simulink model "Dfig2014a"  (R2016a)
settings: Solver=ode45  StartTime=0.0  StopTime=1  RelTol=1e-3
values from neighbouring files (symbols this model uses):
  beta = beta (k)    [Parameter_2M_DFIG.m]    (also in Parameter_2M_DFIG_GSC.m)
  Cbus = 80e-3    (= 0.08)    [Parameter_2M_DFIG.m]    (also in Parameter_2M_DFIG_GSC.m; ini2.m; init.m)
  Cbus_bess = 15e-3    (= 0.015)    [Parameter_2M_DFIG.m]    (also in Parameter_2M_DFIG_GSC.m)
  cp_opt_abs = abs(max(Cp))    [Parameter_2M_DFIG.m]    (also in Parameter_2M_DFIG_GSC.m)
  D = 0.1    [Parameter_2M_DFIG.m]    (also in Parameter_2M_DFIG_GSC.m; ini.m = 0.001; ini2.m = 0.001; init.m = 0.001)
  f = 50    [Parameter_2M_DFIG.m]    (also in Parameter_2M_DFIG_GSC.m = 60; ini.m; ini2.m; init.m)
  Fs = 1.8    [Parameter_2M_DFIG.m]    (also in Parameter_2M_DFIG_GSC.m; ini.m = Vs*sqrt(2/3)/(2*pi*f); ini2.m = Vs*sqrt(2/3)/(2*pi*f); init.m = Vs*sqrt(2/3)/(2*pi*f))
  fsw = 4e3    (= 4000)    [Parameter_2M_DFIG.m]    (also in Parameter_2M_DFIG_GSC.m; ini.m; ini2.m; init.m)
  J = 90    [Parameter_2M_DFIG.m]    (also in Parameter_2M_DFIG_GSC.m; ini.m = 127; ini2.m = 127; init.m = 127)
  ki_id = (wni^2)*Lr*sigma    (= 491.599501999)    [Parameter_2M_DFIG.m]    (also in Parameter_2M_DFIG_GSC.m; ini.m; ini2.m; init.m)
  ki_idg = (wnig^2)*Lg    (= 68.6450725305)    [Parameter_2M_DFIG.m]    (also in Parameter_2M_DFIG_GSC.m; ini2.m = 56.8489213503; init.m = 56.8489213503)
  ki_iq = ki_id    (= 491.599501999)    [Parameter_2M_DFIG.m]    (also in Parameter_2M_DFIG_GSC.m; ini.m; ini2.m; init.m)
  ki_iqg = ki_idg    (= 68.6450725305)    [Parameter_2M_DFIG.m]    (also in Parameter_2M_DFIG_GSC.m; ini2.m = 56.8489213503; init.m = 56.8489213503)
  ki_v = -300000    [Parameter_2M_DFIG.m]    (also in Parameter_2M_DFIG_GSC.m; ini2.m; init.m)
  kp_id = (2*wni*sigma*Lr)-Rr    (= 0.5771)    [Parameter_2M_DFIG.m]    (also in Parameter_2M_DFIG_GSC.m; ini.m; ini2.m; init.m)
  kp_idg = (2*wnig*Lg)-Rg    (= 0.364153420404)    [Parameter_2M_DFIG.m]    (also in Parameter_2M_DFIG_GSC.m; ini2.m = 0.301572894745; init.m = 0.301572894745)
  kp_iq = kp_id    (= 0.5771)    [Parameter_2M_DFIG.m]    (also in Parameter_2M_DFIG_GSC.m; ini.m; ini2.m; init.m)
  kp_iqg = kp_idg    (= 0.364153420404)    [Parameter_2M_DFIG.m]    (also in Parameter_2M_DFIG_GSC.m; ini2.m = 0.301572894745; init.m = 0.301572894745)
  kp_v = -1000    [Parameter_2M_DFIG.m]    (also in Parameter_2M_DFIG_GSC.m; ini2.m; init.m)
  Kpg = 1/(1.5*Vs*sqrt(2/3))    [Parameter_2M_DFIG.m]    (also in Parameter_2M_DFIG_GSC.m; ini2.m; init.m)
  Kqg = -Kpg    [Parameter_2M_DFIG.m]    (also in Parameter_2M_DFIG_GSC.m; ini2.m; init.m)
  lambda_opt = abs(lambda(posicion))    [Parameter_2M_DFIG.m]    (also in Parameter_2M_DFIG_GSC.m)
  Lg = 483e-6    (= 0.000483)    [Parameter_2M_DFIG.m]    (also in Parameter_2M_DFIG_GSC.m; ini2.m = 0.0004; init.m = 0.0004)
  Lg_bess = 600e-6    (= 0.0006)    [Parameter_2M_DFIG.m]    (also in Parameter_2M_DFIG_GSC.m)
  Lm = 2.5e-3    (= 0.0025)    [Parameter_2M_DFIG.m]    (also in Parameter_2M_DFIG_GSC.m; ini.m; ini2.m; init.m)
  Lr = Lm + Lsr    (= 0.002587)    [Parameter_2M_DFIG.m]    (also in Parameter_2M_DFIG_GSC.m; ini.m; ini2.m; init.m)
  Ls = Lm + Lsi    (= 0.002587)    [Parameter_2M_DFIG.m]    (also in Parameter_2M_DFIG_GSC.m; ini.m; ini2.m; init.m)
  Lsi = 87e-6    (= 8.7e-05)    [Parameter_2M_DFIG.m]    (also in Parameter_2M_DFIG_GSC.m; ini.m; ini2.m; init.m)
  N = 100    [Parameter_2M_DFIG.m]    (also in Parameter_2M_DFIG_GSC.m; ini2.m; init.m)
  p = 2    [Parameter_2M_DFIG.m]    (also in Parameter_2M_DFIG_GSC.m; ini.m; ini2.m; init.m)
  Ps = 2e6    (= 2000000)    [Parameter_2M_DFIG.m]    (also in Parameter_2M_DFIG_GSC.m; ini.m; ini2.m; init.m)
  Radio = 44    [Parameter_2M_DFIG.m]    (also in Parameter_2M_DFIG_GSC.m; ini2.m = 42; init.m = 42)
  Rg = 20e-6    (= 2e-05)    [Parameter_2M_DFIG.m]    (also in Parameter_2M_DFIG_GSC.m; ini2.m; init.m)
  Rg_bess = 20e-5    (= 0.0002)    [Parameter_2M_DFIG.m]    (also in Parameter_2M_DFIG_GSC.m)
  ro = 1.225    [Parameter_2M_DFIG.m]    (also in Parameter_2M_DFIG_GSC.m; ini2.m; init.m)
  Rr = 2.9e-3    (= 0.0029)    [Parameter_2M_DFIG.m]    (also in Parameter_2M_DFIG_GSC.m; ini.m; ini2.m; init.m)
  Rs = 2.6e-3    (= 0.0026)    [Parameter_2M_DFIG.m]    (also in Parameter_2M_DFIG_GSC.m; ini.m; ini2.m; init.m)
  sigma = 1- Lm^2/(Ls*Lr)    (= 0.0661284179513)    [Parameter_2M_DFIG.m]    (also in Parameter_2M_DFIG_GSC.m; ini.m; ini2.m; init.m)
  Ts = 1/fsw/f    (= 5e-06)    [Parameter_2M_DFIG.m]    (also in Parameter_2M_DFIG_GSC.m = 4.16666666667e-06; ini.m; ini2.m; init.m)
  Vbus_ref = 1200    [Parameter_2M_DFIG.m]    (also in Parameter_2M_DFIG_GSC.m)
  Vs = 690    [Parameter_2M_DFIG.m]    (also in Parameter_2M_DFIG_GSC.m; ini.m; ini2.m; init.m)
undefined symbols (not defined in the file or in its folder): D1, D11, Delta, DiscIntNeverNeededParam, Ion, Lithium
libraries: powerlib x39, powerlib_meascontrol x10, electricdrivelib x1, sps_avr x1
(part 1 of 2)
settings Model: Creator=admin  LastModifiedBy=UFABC
settings DataIOCC: LimitDataPoints=on  SaveFormat=Array
settings DebuggingCC: UnderspecifiedInitializationDetection=Classic  MergeDetectMultiDrivingBlocksExec=none  SolverPrmCheckMsg=warning  StateNameClashWarn=warning
settings HardwareCC: ProdBitPerPointer=32  ProdLargestAtomicFloat=None  ProdIntDivRoundTo=Undefined  ProdEndianess=Unspecified  ProdWordSize=32  ProdHWDeviceType=32-bit Generic
settings ModelReferenceCC: PropagateSignalLabelsOutOfModel=off
settings ConfigComp: CovModelRefEnable=Off

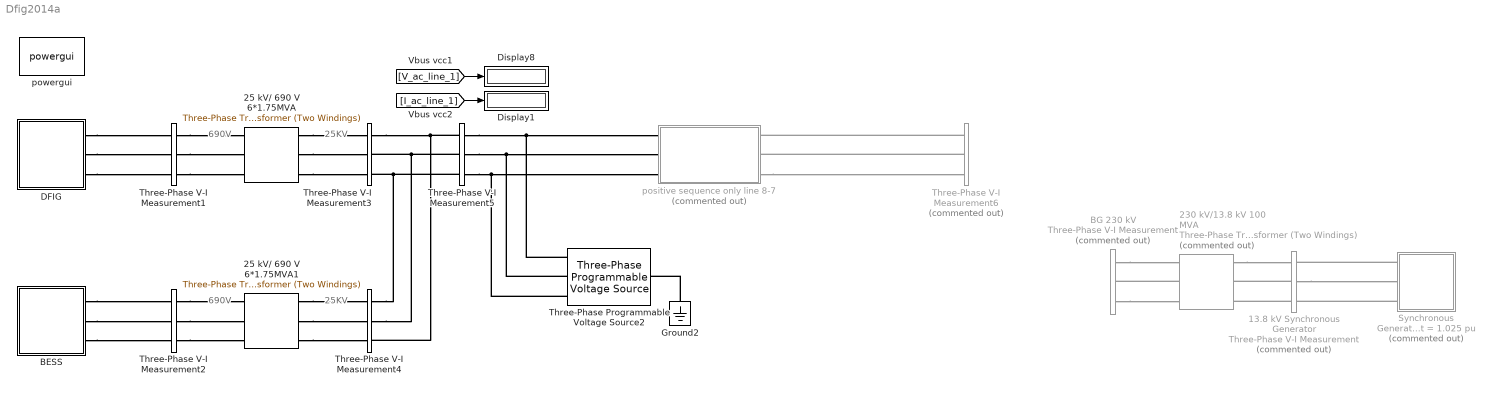
== system Dfig2014a ==
  note: 690V
  note: 25KV
  note: 690V
  note: 25KV
  13.8 kV Synchronous Generator : powerlib/Measurements/Three-Phase V-I Measurement  Commented=on  VoltageMeasurement=phase-to-ground  SetLabelV=on  LabelV=Vabc_GERA  Vpu=on  VpuLL=off  CurrentMeasurement=yes  SetLabelI=on  LabelI=Iabc_GERA  Ipu=on  Pbase=100e6  Vbase=13.8e3  OutputType=Complex  PhasorSimulation=off  PSBequivalent=0
  230 kV/13.8 kV 100 MVA : powerlib/Elements/Three-Phase Transformer (Two Windings)  Commented=on  Winding1Connection=Yg  Winding2Connection=Delta (D1)  CoreType=Three single-phase transformers  SetSaturation=off  Hysteresis=off  DataFile='basic_model'  SetInitialFlux=off  Measurements=None  UNITS=pu  NominalPower=[110e6 60 ]  Winding1="[ 25e3  0   0.0576]"  Winding2="[ 13.8e3  0  0.0576]"  Rm=500  Lm=500  L0=0.5  Saturation="[ 0,0  ;  0.005,1.2  ;  1.0,1.4 ]"  InitialFluxes=[ 0.8 , -0.8 , 0.7 ]  MoreParameters=off  BreakLoop=off  DataType=off  TransfoNumber=0
  25 kV/ 690 V 6*1.75MVA : powerlib/Elements/Three-Phase Transformer (Two Windings)  Winding1Connection=Delta (D11)  Winding2Connection=Yg  CoreType=Three single-phase transformers  SetSaturation=off  Hysteresis=off  DataFile='hysteresis'  SetInitialFlux=off  Measurements=None  UNITS=SI  NominalPower="[2.8e6*6  f]"  Winding1=[25000 0.14881 0.011842]  Winding2=[690 2.624e-05 2.0881e-06]  Rm=89286  Lm=Inf  L0=0.5  Saturation=[0 0;0.47518 112.54;197.99 142.55]  InitialFluxes=[75.026 -75.026 65.648]  MoreParameters=off  BreakLoop=off  DataType=on  TransfoNumber=0
  25 kV/ 690 V 6*1.75MVA1 : powerlib/Elements/Three-Phase Transformer (Two Windings)  Winding1Connection=Delta (D11)  Winding2Connection=Yg  CoreType=Three single-phase transformers  SetSaturation=off  Hysteresis=off  DataFile='hysteresis'  SetInitialFlux=off  Measurements=None  UNITS=SI  NominalPower="[2.8e6*6  f]"  Winding1=[25000 0.14881 0.011842]  Winding2=[690 2.624e-05 2.0881e-06]  Rm=89286  Lm=Inf  L0=0.5  Saturation=[0 0;0.47518 112.54;197.99 142.55]  InitialFluxes=[75.026 -75.026 65.648]  MoreParameters=off  BreakLoop=off  DataType=on  TransfoNumber=0
  BESS : Subsystem
  BG 230 kV : powerlib/Measurements/Three-Phase V-I Measurement  Commented=on  VoltageMeasurement=phase-to-ground  SetLabelV=on  LabelV=Vabc_BG  Vpu=on  VpuLL=off  CurrentMeasurement=yes  SetLabelI=on  LabelI=Iabc_BG  Ipu=on  Pbase=100e6  Vbase=230e3  OutputType=Complex  PhasorSimulation=off  PSBequivalent=0
  DFIG : Subsystem
  Display1 : Display
  Display8 : Display
  Ground2 : powerlib/Elements/Ground  LConnTagsString=a
  Synchronous Generator 100 MVA Vt = 1.025 pu : Subsystem  Commented=on
      mask Display:
      | disp('SG');
      | port_label('LConn', 1, 'A')
      | port_label('LConn', 2, 'B')
      | port_label('LConn', 3, 'C')
  Three-Phase Programmable Voltage Source2 : powerlib/Electrical Sources/Three-Phase Programmable Voltage Source  PositiveSequence="[25e3  0 f]"  VariationEntity=Frequency  VariationType=Table of time-amplitude pairs  VariationTypeAlt=Step  VariationStep=-1.5  VariationRate=1.5  VariationMagnitude=0.3  VariationFrequency=2  VariationTiming=[3 4]  VariationPhaseA=off  Amplitudes=[1 0.8 1.2 1.0]  TimeValues=[0 0.1 0.15 0.2]  HarmonicGeneration=off  HarmonicA=[3 0.2 -25 0]  HarmonicB=[2 0.15 35 2]  Timing="[0.05  3]"  BusType=swing  Pref=0  Qref=0  Qmin=-inf  Qmax=inf
  Three-Phase V-I Measurement1 : powerlib/Measurements/Three-Phase V-I Measurement  VoltageMeasurement=phase-to-ground  SetLabelV=on  LabelV=V_ac_dfig_low  Vpu=off  VpuLL=off  CurrentMeasurement=yes  SetLabelI=on  LabelI=I_ac_dfig_low  Ipu=off  Pbase=100e6  Vbase=500e3  OutputType=Complex  PhasorSimulation=off  PSBequivalent=0
  Three-Phase V-I Measurement2 : powerlib/Measurements/Three-Phase V-I Measurement  VoltageMeasurement=phase-to-ground  SetLabelV=on  LabelV=V_ac_bat_low  Vpu=off  VpuLL=off  CurrentMeasurement=yes  SetLabelI=on  LabelI=I_ac_bat_low  Ipu=off  Pbase=100e6  Vbase=500e3  OutputType=Complex  PhasorSimulation=off  PSBequivalent=0
  Three-Phase V-I Measurement3 : powerlib/Measurements/Three-Phase V-I Measurement  VoltageMeasurement=phase-to-ground  SetLabelV=on  LabelV=V_ac_dfig_H  Vpu=off  VpuLL=off  CurrentMeasurement=yes  SetLabelI=on  LabelI=I_ac_dfig_H  Ipu=off  Pbase=100e6  Vbase=500e3  OutputType=Complex  PhasorSimulation=off  PSBequivalent=0
  Three-Phase V-I Measurement4 : powerlib/Measurements/Three-Phase V-I Measurement  VoltageMeasurement=phase-to-ground  SetLabelV=on  LabelV=V_ac_bat_H  Vpu=off  VpuLL=off  CurrentMeasurement=yes  SetLabelI=on  LabelI=I_ac_bat_H  Ipu=off  Pbase=100e6  Vbase=500e3  OutputType=Complex  PhasorSimulation=off  PSBequivalent=0
  Three-Phase V-I Measurement5 : powerlib/Measurements/Three-Phase V-I Measurement  VoltageMeasurement=phase-to-ground  SetLabelV=on  LabelV=V_ac_line_1  Vpu=off  VpuLL=off  CurrentMeasurement=yes  SetLabelI=on  LabelI=I_ac_line_1  Ipu=off  Pbase=100e6  Vbase=500e3  OutputType=Complex  PhasorSimulation=off  PSBequivalent=0
  Three-Phase V-I Measurement6 : powerlib/Measurements/Three-Phase V-I Measurement  Commented=on  VoltageMeasurement=phase-to-ground  SetLabelV=on  LabelV=V_ac_line_2  Vpu=off  VpuLL=off  CurrentMeasurement=yes  SetLabelI=on  LabelI=I_ac_line_2  Ipu=off  Pbase=100e6  Vbase=500e3  OutputType=Complex  PhasorSimulation=off  PSBequivalent=0
  positive sequence only line 8-7 : Subsystem  Commented=on  mask{Sbase=3, Vbase=25, Fnom=f, R=0.0170, X=0.0920, B=0.0790, l=1}
      mask prompts: Sbase "Base Power (MW)"; Vbase "Base Voltage (kV)"; Fnom "Base Frequency (Hz)"; R "R (pu)"; X "XL (pu)"; B "Bshunt/2 (pu)"; l "Line lenght [1 for total pu values]"
      mask Display:
      | plot(0,0,100,100,[20,20,80,80,90,80,80,20,20,10],[50,40,40,50,50,50,61,61,50,50],[56,39],[55,55],[44,44],[44,55],[53,50,50],[44,48,55])
      | port_label('RConn', 1, 'A')
      | port_label('RConn', 2, 'B')
      | port_label('RConn', 3, 'C')
      | port_label('LConn', 1, 'A')
      | port_label('LConn', 2, 'B')
      | port_label('LConn', 3, 'C')
  powergui : powerlib/powergui  Priority=1  SimulationMode=Discrete  SolverType=Tustin  SampleTime=Ts  frequency=60  SPID=off  DisableSnubberDevices=off  DisableRonSwitches=off  DisableVfSwitches=off  SwTol=0  DisplayEquations=off  Interpol=off  ExternalGateDelay=off  methode=off  Ts=0  FunctionMessages=off  echomessages=off  HookPort=off  EnableUseOfTLC=off  x0status=blocks  frequencyindice=50  Pbase=100e6  ErrMax=1e-4  Iterations=50  UnitsV=kV  UnitsW=MW  buscounter=0  RestoreLinks=warning  ResistiveCurrentMeasurement=off  Frange=[0:2:500]  Ylog=off  Xlog=on  ShowGrid=off  save=off  variable=ZData  structure=0  ZoomFFT=off  StartTime=0.0  cycles=1  DisplayStyle=1  fundamental=60  FreqAxis=off  MaxFrequency=1000  frequencyindicesteady=1  RmsSteady=1  display=off
  wires:
  [V_ac_line_1] -> Display8/1
  [I_ac_line_1] -> Display1/1
  connections:
  BESS/RConn1 -- Three-Phase V-I Measurement2/LConn1
  BESS/RConn2 -- Three-Phase V-I Measurement2/LConn2
  BESS/RConn3 -- Three-Phase V-I Measurement2/LConn3
  DFIG/RConn3 -- Three-Phase V-I Measurement1/LConn3
  DFIG/RConn1 -- Three-Phase V-I Measurement1/LConn1
  DFIG/RConn2 -- Three-Phase V-I Measurement1/LConn2
  Ground2/LConn1 -- Three-Phase Programmable Voltage Source2/LConn1
  Three-Phase V-I Measurement1/RConn1 -- 25 kV/ 690 V 6*1.75MVA/RConn1
  Three-Phase V-I Measurement1/RConn2 -- 25 kV/ 690 V 6*1.75MVA/RConn2
  Three-Phase V-I Measurement1/RConn3 -- 25 kV/ 690 V 6*1.75MVA/RConn3
  25 kV/ 690 V 6*1.75MVA/LConn1 -- Three-Phase V-I Measurement3/LConn1
  25 kV/ 690 V 6*1.75MVA/LConn2 -- Three-Phase V-I Measurement3/LConn2
  25 kV/ 690 V 6*1.75MVA/LConn3 -- Three-Phase V-I Measurement3/LConn3
  25 kV/ 690 V 6*1.75MVA1/LConn1 -- Three-Phase V-I Measurement4/LConn1
  25 kV/ 690 V 6*1.75MVA1/LConn2 -- Three-Phase V-I Measurement4/LConn2
  25 kV/ 690 V 6*1.75MVA1/LConn3 -- Three-Phase V-I Measurement4/LConn3
  Three-Phase V-I Measurement2/RConn1 -- 25 kV/ 690 V 6*1.75MVA1/RConn1
  Three-Phase V-I Measurement2/RConn2 -- 25 kV/ 690 V 6*1.75MVA1/RConn2
  Three-Phase V-I Measurement2/RConn3 -- 25 kV/ 690 V 6*1.75MVA1/RConn3
  BG 230 kV/LConn1 -- 230 kV/13.8 kV 100 MVA/LConn1
  230 kV/13.8 kV 100 MVA/LConn2 -- BG 230 kV/LConn2
  13.8 kV Synchronous Generator/RConn2 -- 230 kV/13.8 kV 100 MVA/RConn2
  13.8 kV Synchronous Generator/RConn3 -- 230 kV/13.8 kV 100 MVA/RConn3
  13.8 kV Synchronous Generator/LConn2 -- Synchronous Generator 100 MVA Vt = 1.025 pu/LConn2
  Synchronous Generator 100 MVA Vt = 1.025 pu/LConn3 -- 13.8 kV Synchronous Generator/LConn3
  230 kV/13.8 kV 100 MVA/RConn1 -- 13.8 kV Synchronous Generator/RConn1
  BG 230 kV/LConn3 -- 230 kV/13.8 kV 100 MVA/LConn3
  Synchronous Generator 100 MVA Vt = 1.025 pu/LConn1 -- 13.8 kV Synchronous Generator/LConn1
  Three-Phase V-I Measurement3/RConn1 -- Three-Phase V-I Measurement5/LConn1 -- Three-Phase V-I Measurement4/RConn3
  Three-Phase V-I Measurement4/RConn2 -- Three-Phase V-I Measurement3/RConn2 -- Three-Phase V-I Measurement5/LConn2
  Three-Phase V-I Measurement4/RConn1 -- Three-Phase V-I Measurement5/LConn3 -- Three-Phase V-I Measurement3/RConn3
  Three-Phase V-I Measurement5/RConn1 -- Three-Phase Programmable Voltage Source2/RConn1 -- positive sequence only line 8-7/RConn1
  Three-Phase V-I Measurement5/RConn2 -- Three-Phase Programmable Voltage Source2/RConn2 -- positive sequence only line 8-7/RConn2
  Three-Phase V-I Measurement5/RConn3 -- Three-Phase Programmable Voltage Source2/RConn3 -- positive sequence only line 8-7/RConn3
  Three-Phase V-I Measurement6/LConn1 -- positive sequence only line 8-7/LConn1
  Three-Phase V-I Measurement6/LConn2 -- positive sequence only line 8-7/LConn2
  positive sequence only line 8-7/LConn3 -- Three-Phase V-I Measurement6/LConn3

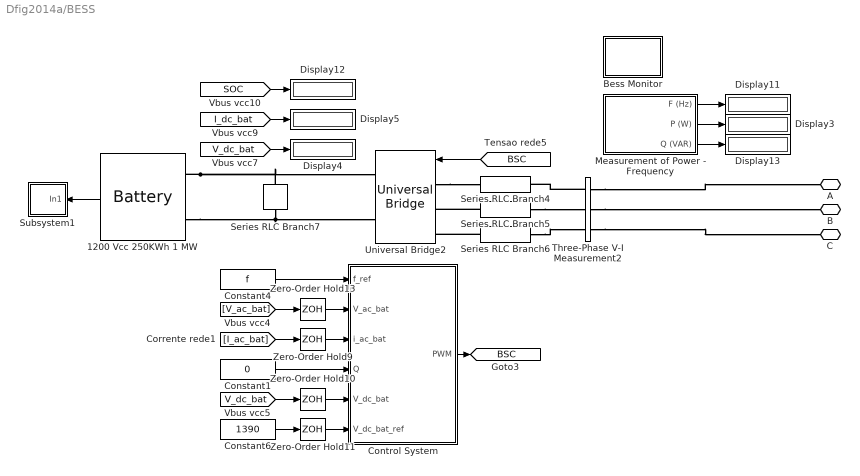
== system Dfig2014a/BESS ==
  "1200 Vcc 250KWh 1 MW " : electricdrivelib/Extra Sources/Battery  BatType=Lithium-Ion  ShowTempParam=off  ThermalPreset=no  NomV=1200  NomQ=100  SOC=71.5  Batt_Tr=30  PresetModel=on  MaxQ=100  MinV=900  FullV=1396.7846  Dis_rate=43.4783  R=0.12  Normal_OP=90.4348  expZone="[1296.463      4.9130435]"  current=[6.5 13 32.5]  Units=Time  Tci=20  NomT=25  T2=0  MaxQ2=2.208  FullV2=3.45  Normal_OP2=2.8  expZone2="[3.22        0.23]"  Rca=0.6  ti=1000  Dp=0
  Bess Monitor : Subsystem
  Constant1 : Constant  Value=0
  Constant4 : Constant  Value=f
  Constant6 : Constant  Value=1390
  Control System : Subsystem
  Display{3..5,11..13} (6 alike) : Display
  Measurement of Power - Frequency : Subsystem
  Series RLC Branch4 : powerlib/Elements/Series RLC Branch  LConnTagsString=__new0  RConnTagsString=__new0  BranchType=RL  Resistance=Rg_bess  Inductance=Lg_bess  SetiL0=off  InitialCurrent=0  Capacitance=0  Setx0=off  InitialVoltage=0  Measurements=None
  Series RLC Branch5 : powerlib/Elements/Series RLC Branch  LConnTagsString=__new0  RConnTagsString=__new0  BranchType=RL  Resistance=Rg_bess  Inductance=Lg_bess  SetiL0=off  InitialCurrent=0  Capacitance=0  Setx0=off  InitialVoltage=0  Measurements=None
  Series RLC Branch6 : powerlib/Elements/Series RLC Branch  LConnTagsString=__new0  RConnTagsString=__new0  BranchType=RL  Resistance=Rg_bess  Inductance=Lg_bess  SetiL0=off  InitialCurrent=0  Capacitance=0  Setx0=off  InitialVoltage=0  Measurements=None
  Series RLC Branch7 : powerlib/Elements/Series RLC Branch  LConnTagsString=__new0  RConnTagsString=__new0  BranchType=C  Resistance=1  Inductance=1e-3  SetiL0=off  InitialCurrent=0  Capacitance=Cbus_bess  Setx0=off  InitialVoltage=0  Measurements=Branch voltage
  Subsystem1 : Subsystem
  Three-Phase V-I Measurement2 : powerlib/Measurements/Three-Phase V-I Measurement  VoltageMeasurement=phase-to-ground  SetLabelV=on  LabelV=V_ac_bat  Vpu=off  VpuLL=off  CurrentMeasurement=yes  SetLabelI=on  LabelI=I_ac_bat  Ipu=off  Pbase=100e6  Vbase=500e3  OutputType=Complex  PhasorSimulation=off  PSBequivalent=0
  Universal Bridge2 : powerlib/Power Electronics/Universal Bridge  Arms=3  SnubberResistance=1e5  SnubberCapacitance=inf  Device=Ideal Switches  Ron=1e-3  Lon=0  ForwardVoltages="[  0  0  ]"  ForwardVoltage=0  GTOparameters=[ 10e-6 , 20e-6 ]  IGBTparameters=[ 1e-6 , 2e-6 ]  Measurements=None  Measurements_2=None  converterType=Rectifier
  Zero-Order Hold{9..11,13} (4 alike) : ZeroOrderHold  SampleTime=1/fsw
  A : PMIOPort  Port=1  Side=Right
  B : PMIOPort  Port=2  Side=Right
  C : PMIOPort  Port=3  Side=Right
  tag scope: BSC=global
  wires:
  Zero-Order Hold10/1 -> Control System/5(V_dc_bat)
  Constant4/1 -> Control System/1(f_ref)
  [V_dc_bat] -> Zero-Order Hold10/1
  [I_dc_bat] -> Display5/1
  Control System/1(PWM) -> [BSC]
  Zero-Order Hold11/1 -> Control System/6(V_dc_bat_ref)
  [V_dc_bat] -> Display4/1
  "1200 Vcc 250KWh 1 MW "/1 -> Subsystem1/1(In1)
  Zero-Order Hold13/1 -> Control System/2("V_ac_bat ")
  [V_ac_bat] -> Zero-Order Hold13/1
  Constant6/1 -> Zero-Order Hold11/1
  Zero-Order Hold9/1 -> Control System/3(i_ac_bat)
  [BSC] -> Universal Bridge2/1
  Constant1/1 -> Control System/4(Q)
  [I_ac_bat] -> Zero-Order Hold9/1
  Measurement of Power - Frequency/2(P (W)) -> Display3/1
  Measurement of Power - Frequency/1(F (Hz)) -> Display11/1
  Measurement of Power - Frequency/3(Q (VAR)) -> Display13/1
  [SOC] -> Display12/1
  connections:
  Series RLC Branch7/RConn1 -- "1200 Vcc 250KWh 1 MW "/LConn2 -- Universal Bridge2/RConn2
  "1200 Vcc 250KWh 1 MW "/LConn1 -- Series RLC Branch7/LConn1 -- Universal Bridge2/RConn1
  Universal Bridge2/LConn1 -- Series RLC Branch4/LConn1
  Three-Phase V-I Measurement2/LConn1 -- Series RLC Branch4/RConn1
  Series RLC Branch6/LConn1 -- Universal Bridge2/LConn3
  Series RLC Branch5/RConn1 -- Three-Phase V-I Measurement2/LConn2
  Series RLC Branch5/LConn1 -- Universal Bridge2/LConn2
  Series RLC Branch6/RConn1 -- Three-Phase V-I Measurement2/LConn3
  Three-Phase V-I Measurement2/RConn1 -- A/RConn1
  Three-Phase V-I Measurement2/RConn2 -- B/RConn1
  Three-Phase V-I Measurement2/RConn3 -- C/RConn1

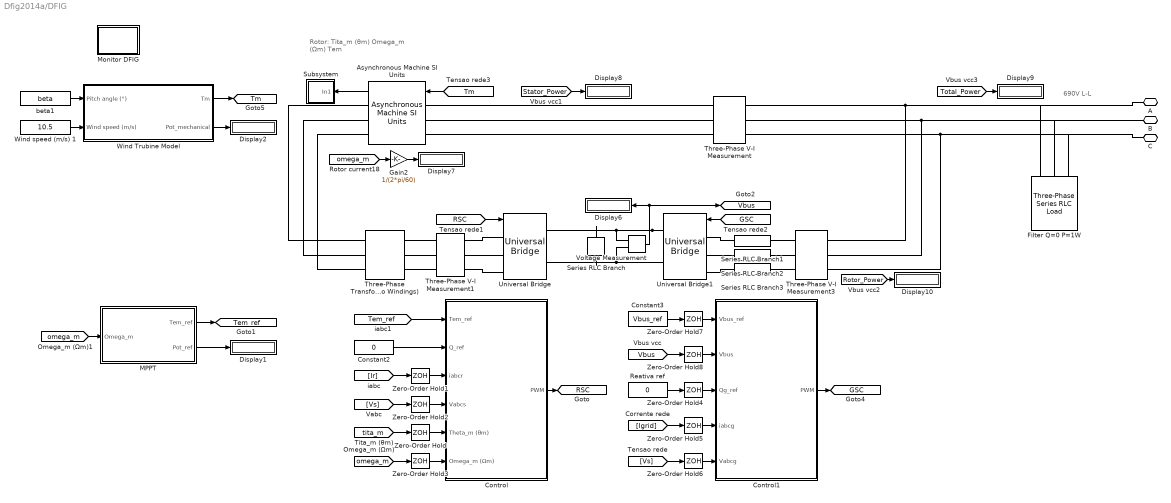
== system Dfig2014a/DFIG ==
  note: 690V L-L
  note: Rotor:
      | Tita_m (θm)
      | Omega_m (Ωm)
      | Tem
  Asynchronous Machine SI Units : powerlib/Machines/Asynchronous Machine SI Units  RotorType=Wound  PresetModel=No  MechanicalLoad=Torque Tm  ShowDetailedParameters=on  ReferenceFrame=Rotor  Units=SI  MeasurementBus=off  NominalParameters=[ Ps Vs f ]  Stator=[ Rs , Lsi]  Rotor=[ Rr , Lsi]  Cage1=[ 0.022 0.226/377]  Cage2=[ 0.022 0.226/377]  Lm=Lm  Mechanical=[ J D 2 ]  PolePairs=2  InitialConditions=[1 0 0 0 0 0 0 0]  SimulateSaturation=off  Saturation=[14.03593122, 27.81365428, 53.79336849, 72.68890987, 97.98006896, 148.6815601, 215.7428561, 302.9841135, 420.4778367 ; 230, 322, 414, 460, 506, 552, 598, 644, 690]  LoadFlowParameters=1492000  TsPowergui=0  TsBlock=-1  IterativeModel=Trapezoidal non iterative  IterativeDiscreteModel=Trapezoidal non iterative  Pmec=0
  Constant2 : Constant  Value=0
  Constant3 : Constant  Value=Vbus_ref
  Control : Subsystem
  Control1 : Subsystem
  Display{1..2,6..10} (7 alike) : Display
  Filter Q=0 P=1W : powerlib/Elements/Three-Phase Series RLC Load  LConnTagsString=A|B|C  Configuration=Y (grounded)  NominalVoltage=Vs  Vabc=[1e3 1e3 1e3]  Vabcp=[1e3 1e3 1e3]  NominalFrequency=f  UnbalancedPower=off  ActivePower=1  InductivePower=0  CapacitivePower=0  Pabc=[10e3 9e3 11e3]  QLabc=[100 90 110]  QCabc=[100 90 110]  Pabcp=[10e3 9e3 11e3]  QLabcp=[100 90 110]  QCabcp=[100 90 110]  Measurements=None  LoadType=constant Z
  Gain2 : Gain  Gain=1/(2*pi/60)
  MPPT : Subsystem
  Monitor DFIG : Subsystem
  Reativa ref : Constant  Value=0
  Series RLC Branch : powerlib/Elements/Series RLC Branch  LConnTagsString=__new0  RConnTagsString=__new0  BranchType=C  Resistance=1  Inductance=1e-3  SetiL0=off  InitialCurrent=0  Capacitance=Cbus  Setx0=off  InitialVoltage=0  Measurements=Branch voltage
  Series RLC Branch1 : powerlib/Elements/Series RLC Branch  LConnTagsString=__new0  RConnTagsString=__new0  BranchType=RL  Resistance=Rg  Inductance=Lg  SetiL0=off  InitialCurrent=0  Capacitance=0  Setx0=off  InitialVoltage=0  Measurements=None
  Series RLC Branch2 : powerlib/Elements/Series RLC Branch  LConnTagsString=__new0  RConnTagsString=__new0  BranchType=RL  Resistance=Rg  Inductance=Lg  SetiL0=off  InitialCurrent=0  Capacitance=0  Setx0=off  InitialVoltage=0  Measurements=None
  Series RLC Branch3 : powerlib/Elements/Series RLC Branch  LConnTagsString=__new0  RConnTagsString=__new0  BranchType=RL  Resistance=Rg  Inductance=Lg  SetiL0=off  InitialCurrent=0  Capacitance=0  Setx0=off  InitialVoltage=0  Measurements=None
  Subsystem : Subsystem
  Three-Phase Transformer (Two Windings) : powerlib/Elements/Three-Phase Transformer (Two Windings)  Winding1Connection=Y  Winding2Connection=Y  CoreType=Three single-phase transformers  SetSaturation=off  Hysteresis=off  DataFile='hysteresis'  SetInitialFlux=off  Measurements=None  UNITS=SI  NominalPower=[ Ps , f]  Winding1=[Vs 0 0]  Winding2=[Vs/u 0 0]  Rm=1.0805e+06  Lm=2866  L0=0.5  Saturation=[0 0;0.66653 1910.3;277.72 2419.7]  InitialFluxes=[1273.5 -1273.5 1114.3]  MoreParameters=off  BreakLoop=off  DataType=on  TransfoNumber=1
  Three-Phase V-I Measurement : powerlib/Measurements/Three-Phase V-I Measurement  VoltageMeasurement=phase-to-ground  SetLabelV=on  LabelV=Vs  Vpu=off  VpuLL=off  CurrentMeasurement=yes  SetLabelI=on  LabelI=Is  Ipu=off  Pbase=100e6  Vbase=500e3  OutputType=Complex  PhasorSimulation=off  PSBequivalent=0
  Three-Phase V-I Measurement1 : powerlib/Measurements/Three-Phase V-I Measurement  VoltageMeasurement=phase-to-phase  SetLabelV=on  LabelV=Vr  Vpu=off  VpuLL=off  CurrentMeasurement=yes  SetLabelI=on  LabelI=Ir  Ipu=off  Pbase=100e6  Vbase=500e3  OutputType=Complex  PhasorSimulation=off  PSBequivalent=0
  Three-Phase V-I Measurement3 : powerlib/Measurements/Three-Phase V-I Measurement  VoltageMeasurement=phase-to-ground  SetLabelV=on  LabelV=Vgrid  Vpu=off  VpuLL=off  CurrentMeasurement=yes  SetLabelI=on  LabelI=Igrid  Ipu=off  Pbase=100e6  Vbase=500e3  OutputType=Complex  PhasorSimulation=off  PSBequivalent=0
  Universal Bridge : powerlib/Power Electronics/Universal Bridge  Arms=3  SnubberResistance=1e5  SnubberCapacitance=inf  Device=Ideal Switches  Ron=1e-3  Lon=0  ForwardVoltages="[  0  0  ]"  ForwardVoltage=0  GTOparameters=[ 10e-6 , 20e-6 ]  IGBTparameters=[ 1e-6 , 2e-6 ]  Measurements=None  Measurements_2=None  converterType=Rectifier
  Universal Bridge1 : powerlib/Power Electronics/Universal Bridge  Arms=3  SnubberResistance=1e5  SnubberCapacitance=inf  Device=Ideal Switches  Ron=1e-3  Lon=0  ForwardVoltages="[  0  0  ]"  ForwardVoltage=0  GTOparameters=[ 10e-6 , 20e-6 ]  IGBTparameters=[ 1e-6 , 2e-6 ]  Measurements=None  Measurements_2=None  converterType=Rectifier
  Voltage Measurement : powerlib/Measurements/Voltage Measurement  PhasorSimulation=off  OutputType=Complex  PSBequivalent=0
  Wind Trubine Model : Subsystem
  Wind speed (m/s) 1 : Constant  Value=10.5
  Zero-Order Hold{,1..8} (9 alike) : ZeroOrderHold  SampleTime=1/fsw
  beta1 : Constant  Value=beta
  A : PMIOPort  Port=1  Side=Right
  B : PMIOPort  Port=2  Side=Right
  C : PMIOPort  Port=3  Side=Right
  tag scope: GSC=global, RSC=global, Tem_ref=global, Tm=global, Vbus=global
  wires:
  [Igrid] -> Zero-Order Hold5/1
  beta1/1 -> Wind Trubine Model/1(Pitch angle (°))
  Constant3/1 -> Zero-Order Hold7/1
  MPPT/1(Tem_ref) -> [Tem_ref]
  Wind Trubine Model/1(Tm) -> [Tm]
  [Stator_Power] -> Display8/1
  [Tm] -> Asynchronous Machine SI Units/1
  MPPT/2("Pot_ref ") -> Display1/1
  Reativa ref/1 -> Zero-Order Hold4/1
  [GSC] -> Universal Bridge1/1
  Wind Trubine Model/2(Pot_mechanical) -> Display2/1
  [omega_m] -> MPPT/1(Omega_m)
  Control/1(PWM) -> [RSC]
  Wind speed (m/s) 1/1 -> Wind Trubine Model/2(Wind speed (m/s))
  [tita_m] -> Zero-Order Hold/1
  [Tem_ref] -> Control/1(Tem_ref)
  [Rotor_Power] -> Display10/1
  [omega_m] -> Gain2/1
  [Vs] -> Zero-Order Hold2/1
  Asynchronous Machine SI Units/1 -> Subsystem/1(In1)
  Zero-Order Hold/1 -> Control/5(Theta_m (θm))
  Zero-Order Hold2/1 -> Control/4(Vabcs)
  [omega_m] -> Zero-Order Hold3/1
  Gain2/1 -> Display7/1
  Zero-Order Hold1/1 -> Control/3(iabcr)
  Constant2/1 -> Control/2(Q_ref)
  [Vbus] -> Zero-Order Hold8/1
  Zero-Order Hold7/1 -> Control1/1(Vbus_ref)
  [RSC] -> Universal Bridge/1
  Zero-Order Hold3/1 -> Control/6("Omega_m (Ωm) ")
  [Ir] -> Zero-Order Hold1/1
  [Vs] -> Zero-Order Hold6/1
  [Total_Power] -> Display9/1
  Zero-Order Hold6/1 -> Control1/5("Vabcg ")
  Zero-Order Hold5/1 -> Control1/4(iabcg)
  Voltage Measurement/1 -> Display6/1, [Vbus]
  Zero-Order Hold4/1 -> Control1/3(Qg_ref)
  Control1/1(PWM) -> [GSC]
  Zero-Order Hold8/1 -> Control1/2(Vbus)
  connections:
  Three-Phase V-I Measurement/RConn2 -- Filter Q=0 P=1W/LConn2 -- B/RConn1 -- Three-Phase V-I Measurement3/RConn2
  Three-Phase V-I Measurement/RConn1 -- A/RConn1 -- Filter Q=0 P=1W/LConn1 -- Three-Phase V-I Measurement3/RConn1
  Voltage Measurement/LConn2 -- Universal Bridge1/RConn2 -- Universal Bridge/RConn2 -- Series RLC Branch/RConn1
  Universal Bridge1/RConn1 -- Voltage Measurement/LConn1 -- Universal Bridge/RConn1 -- Series RLC Branch/LConn1
  Three-Phase V-I Measurement/RConn3 -- Filter Q=0 P=1W/LConn3 -- C/RConn1 -- Three-Phase V-I Measurement3/RConn3
  Three-Phase Transformer (Two Windings)/LConn2 -- Asynchronous Machine SI Units/RConn2
  Three-Phase Transformer (Two Windings)/LConn3 -- Asynchronous Machine SI Units/RConn3
  Three-Phase V-I Measurement3/LConn2 -- Series RLC Branch2/RConn1
  Three-Phase V-I Measurement1/LConn1 -- Universal Bridge/LConn1
  Three-Phase V-I Measurement/LConn1 -- Asynchronous Machine SI Units/LConn1
  Three-Phase V-I Measurement3/LConn3 -- Series RLC Branch3/RConn1
  Three-Phase Transformer (Two Windings)/LConn1 -- Asynchronous Machine SI Units/RConn1
  Three-Phase V-I Measurement/LConn3 -- Asynchronous Machine SI Units/LConn3
  Three-Phase V-I Measurement3/LConn1 -- Series RLC Branch1/RConn1
  Three-Phase Transformer (Two Windings)/RConn3 -- Three-Phase V-I Measurement1/RConn3
  Three-Phase V-I Measurement1/LConn3 -- Universal Bridge/LConn3
  Universal Bridge1/LConn1 -- Series RLC Branch1/LConn1
  Three-Phase V-I Measurement1/LConn2 -- Universal Bridge/LConn2
  Three-Phase Transformer (Two Windings)/RConn2 -- Three-Phase V-I Measurement1/RConn2
  Universal Bridge1/LConn3 -- Series RLC Branch3/LConn1
  Three-Phase V-I Measurement/LConn2 -- Asynchronous Machine SI Units/LConn2
  Universal Bridge1/LConn2 -- Series RLC Branch2/LConn1
  Three-Phase Transformer (Two Windings)/RConn1 -- Three-Phase V-I Measurement1/RConn1

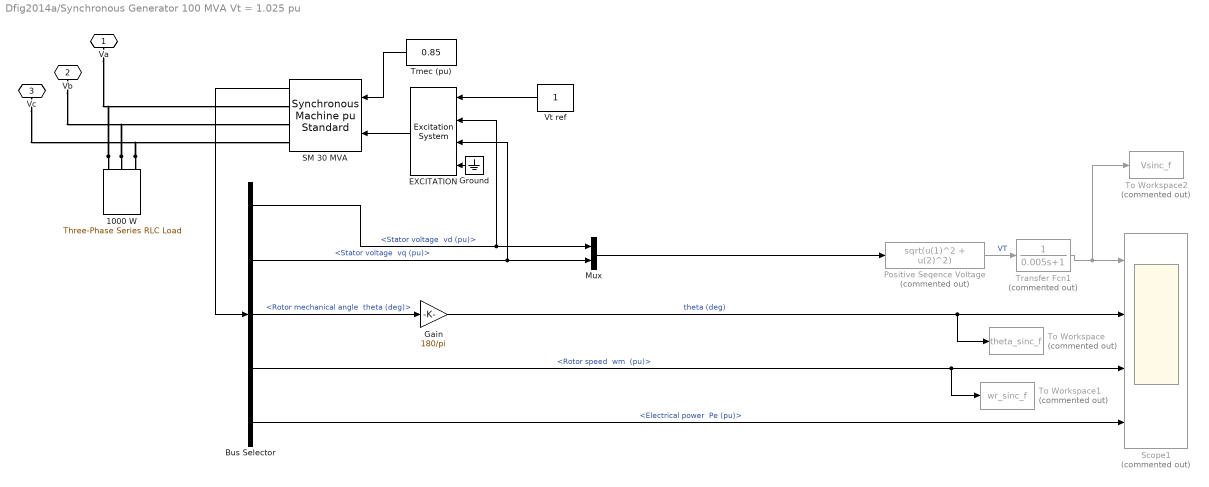
== system Dfig2014a/Synchronous Generator 100 MVA Vt = 1.025 pu ==
  1000 W : powerlib/Elements/Three-Phase Series RLC Load  LConnTagsString=A|B|C  Configuration=Y (grounded)  NominalVoltage=13800  Vabc=[1e3 1e3 1e3]  Vabcp=[1e3 1e3 1e3]  NominalFrequency=60  UnbalancedPower=off  ActivePower=8e6  InductivePower=0  CapacitivePower=0  Pabc=[10e3 9e3 11e3]  QLabc=[100 90 110]  QCabc=[100 90 110]  Pabcp=[10e3 9e3 11e3]  QLabcp=[100 90 110]  QCabcp=[100 90 110]  Measurements=None  LoadType=constant Z
  Bus Selector : BusSelector  OutputSignals="dq0 components.Stator voltage  vd (pu),dq0 components.Stator voltage  vq (pu),Mechanical.Rotor mechanical angle  theta (deg),Mechanical.Rotor speed  wm  (pu),Mechanical.Electrical power  Pe (pu)"
  EXCITATION : sps_avr/Excitation System  tr=0.005  reg=[270, 0.1 ]  exc=[ 1, 0.65 ]  tgr=[ 0, 0 ]  damp=[ 0.048, 0.95 ]  sat=[ 0, 0 ]  lim=[ -4, 7, 0 ]  v0=[1,1.67677]
  Gain : Gain  Gain=180/pi  SaturateOnIntegerOverflow=on  OutDataTypeStr=Inherit: Same as input  ParamDataTypeStr=Inherit: Same as input
  Ground : Ground
  Mux : Mux  Inputs=2
  Positive Seqence Voltage : Fcn  Commented=on  Expr=sqrt(u(1)^2 + u(2)^2)
  SM 30 MVA : powerlib/Machines/Synchronous Machine pu Standard  PresetModel=No  MechanicalLoad=Mechanical power Pm  ShowDetailedParameters=on  RotorType=Salient-pole  Units=per unit standard parameters  MeasurementBus=off  NominalParameters="[ 100e6  13800  60 ]"  Reactances1=[ 1.4 0.231 0.118 1.372 0.8 0.118 0.05 ]  Reactances2="[ 1.3125  0.1813  0.13  1.2578  0.10  0.005 ]"  dAxisTimeConstants=Open-circuit  qAxisTimeConstants=Open-circuit  TimeConstants1="[5.89  0.04 0.099]"  TimeConstants2=[5.5 0.05 1.25 0.19]  TimeConstants3=[]  TimeConstants4=[]  TimeConstants5=[ 3.7, 0.05, 0.05 ]  TimeConstants6=[]  TimeConstants7=[]  TimeConstants8=[]  StatorResistance=0.0031  Mechanical="[3.01  0  20 ]"  PolePairs=20  InitialConditions=[0 -91.23 0.819229 0.819229 0.819229 -55.1025 -175.102 64.8975 1.67677]  SetSaturation=off  Saturation=[0.211 0.418 1.0 1.72 3.35 ; 0.25 0.50 1.0 1.2 1.4]  LoadFlowParameters=[1 80000000 13800 0 0]  TsPowergui=0  TsBlock=-1  IterativeModel=Trapezoidal non iterative  IterativeDiscreteModel=Trapezoidal non iterative  BusType=PV  Pref=0  Qref=0  Qmin=-inf  Qmax=inf  PLF=0  QLF=0
  Scope1 : Scope  Commented=on  NumInputPorts=4
  Tmec (pu) : Constant  Value=0.85
  To Workspace : ToWorkspace  Commented=on  VariableName=theta_sinc_f  SampleTime=-1
      settings: Decimation=dec
  To Workspace1 : ToWorkspace  Commented=on  VariableName=wr_sinc_f  SampleTime=-1
      settings: Decimation=dec
  To Workspace2 : ToWorkspace  Commented=on  VariableName=Vsinc_f  SampleTime=-1
      settings: Decimation=dec
  Transfer Fcn1 : TransferFcn  Commented=on  Denominator=[0.005 1]
  Vt ref : Constant
  Va : PMIOPort  Port=1  Side=Left
  Vb : PMIOPort  Port=2  Side=Left
  Vc : PMIOPort  Port=3  Side=Left
  wires:
  Positive Seqence Voltage/1 -> Transfer Fcn1/1  "VT"
  Gain/1 -> Scope1/2, To Workspace/1  "theta (deg)"
  EXCITATION/1 -> SM 30 MVA/2
  Ground/1 -> EXCITATION/4
  SM 30 MVA/1 -> Bus Selector/1
  Mux/1 -> Positive Seqence Voltage/1
  Bus Selector/4 -> To Workspace1/1, Scope1/3  "<Rotor speed  wm  (pu)>"
  Vt ref/1 -> EXCITATION/1
  Tmec (pu)/1 -> SM 30 MVA/1
  Bus Selector/3 -> Gain/1  "<Rotor mechanical angle  theta (deg)>"
  Transfer Fcn1/1 -> To Workspace2/1, Scope1/1
  Bus Selector/5 -> Scope1/4  "<Electrical power  Pe (pu)>"
  Bus Selector/1 -> EXCITATION/2, Mux/1  "<Stator voltage  vd (pu)>"
  Bus Selector/2 -> EXCITATION/3, Mux/2  "<Stator voltage  vq (pu)>"
  connections:
  1000 W/LConn1 -- SM 30 MVA/RConn1 -- Va/RConn1
  1000 W/LConn2 -- SM 30 MVA/RConn2 -- Vb/RConn1
  1000 W/LConn3 -- SM 30 MVA/RConn3 -- Vc/RConn1

== system Dfig2014a/positive sequence only line 8-7 ==
  Ground1 : powerlib/Elements/Ground  LConnTagsString=a
  Three-Phase Series RLC Branch : powerlib/Elements/Three-Phase Series RLC Branch  LConnTagsString=A|B|C  RConnTagsString=A|B|C  BranchType=RL  Resistance=R*l*((Vbase*1e3)^2/(Sbase*1e6))  Inductance=X*l*((Vbase*1e3)^2/(Sbase*1e6))/(2*pi*Fnom)  Capacitance=1.0  Measurements=None
  Three-Phase Series RLC Branch1 : powerlib/Elements/Three-Phase Series RLC Branch  LConnTagsString=A|B|C  RConnTagsString=A|B|C  BranchType=C  Resistance=5.29  Inductance=119.27e-3  Capacitance=((B*l)/((Vbase*1e3)^2/(Sbase*1e6)))/(2*pi*Fnom)  Measurements=None
  Three-Phase Series RLC Branch2 : powerlib/Elements/Three-Phase Series RLC Branch  LConnTagsString=A|B|C  RConnTagsString=A|B|C  BranchType=C  Resistance=5.29  Inductance=119.27e-3  Capacitance=((B*l)/((Vbase*1e3)^2/(Sbase*1e6)))/(2*pi*Fnom)  Measurements=None
  A : PMIOPort  Port=1  Side=Left
  B : PMIOPort  Port=2  Side=Left
  C : PMIOPort  Port=3  Side=Left
  a : PMIOPort  Port=4  Side=Right
  b : PMIOPort  Port=5  Side=Right
  c : PMIOPort  Port=6  Side=Right
  connections:
  Three-Phase Series RLC Branch1/RConn3 -- Ground1/LConn1 -- Three-Phase Series RLC Branch2/RConn3 -- Three-Phase Series RLC Branch1/RConn1 -- Three-Phase Series RLC Branch2/RConn2 -- Three-Phase Series RLC Branch1/RConn2 -- Three-Phase Series RLC Branch2/RConn1
  Three-Phase Series RLC Branch2/LConn3 -- c/RConn1 -- Three-Phase Series RLC Branch/RConn3
  Three-Phase Series RLC Branch2/LConn2 -- b/RConn1 -- Three-Phase Series RLC Branch/RConn2
  Three-Phase Series RLC Branch2/LConn1 -- a/RConn1 -- Three-Phase Series RLC Branch/RConn1
  Three-Phase Series RLC Branch1/LConn3 -- Three-Phase Series RLC Branch/LConn3 -- C/RConn1
  Three-Phase Series RLC Branch1/LConn2 -- Three-Phase Series RLC Branch/LConn2 -- B/RConn1
  Three-Phase Series RLC Branch1/LConn1 -- Three-Phase Series RLC Branch/LConn1 -- A/RConn1

== system Dfig2014a/BESS/Bess Monitor ==
  note: BATTERY STORAGE SYSTEM
  note: Tip Speed Ratio
  note: Charging Power
  note: Discharging Power
  note: Id current control
  Mux{,13..15} (4 alike) : Mux  Inputs=2
  Scope3 : Scope  NumInputPorts=6
  wires:
  [P_bat_ref] -> Mux14/1
  [V_dc_bat] -> Mux/2
  Mux13/1 -> Scope3/2  "Charging Power (W)"
  [P_SOC_ref] -> Mux13/1
  [P_bat] -> Mux14/2, Mux13/2
  [id_bat_ref] -> Mux15/1
  [V_dc_bat_ref] -> Mux/1
  Mux/1 -> Scope3/1  "Vbus* / Vbus (V)"
  [id_bat] -> Mux15/2
  Mux14/1 -> Scope3/3  "Discharging Power (W)"
  [SOC] -> Scope3/5  "SOC (%)"
  [I_dc_bat] -> Scope3/4  "Battery Current (Amp)"
  Mux15/1 -> Scope3/6  "Id*/Id (Amp)"

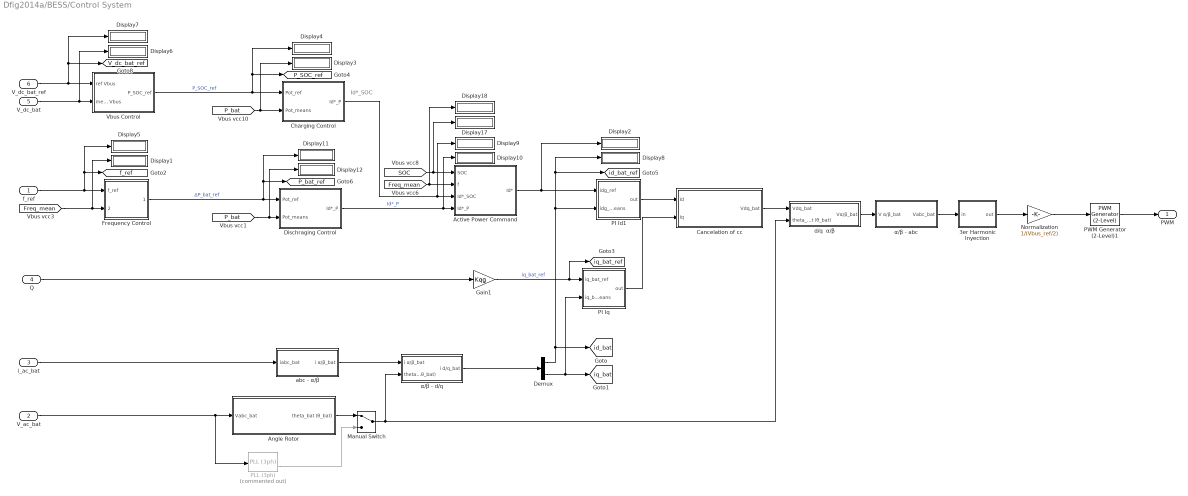
== system Dfig2014a/BESS/Control System ==
  note: Id*_SOC
  f_ref : Inport
  "V_ac_bat " : Inport  Port=2
  i_ac_bat : Inport  Port=3
  Q : Inport  Port=4
  V_dc_bat : Inport  Port=5
  V_dc_bat_ref : Inport  Port=6
  " Angle Rotor" : Subsystem
  3er Harmonic Inyection : Subsystem
  Active Power Command : Subsystem
  Cancelation of cc : Subsystem
  Charging Control : Subsystem
  Demux : Demux  Outputs=2
  Dischraging Control : Subsystem
  Display{1..12,17..18} (14 alike) : Display
  Frequency Control : Subsystem
  Gain1 : Gain  Gain=Kqg
  Manual Switch : ManualSwitch
  Normalization : Gain  Gain=1/(Vbus_ref/2)
  PI Id1 : Subsystem
  PI Iq : Subsystem
  PLL (3ph) : powerlib_meascontrol/PLL/PLL (3ph)  Commented=on  Fmin=45  Par_Init=[0, 60]  ParK=[180, 3200, 1]  TcD=1e-4  MaxRateChangeFreq=12  FilterCutOffFreq=25  Ts=0  AGC=on
      link override Model/abc to dq0: Alignment=Aligned with phase A axis
  PWM Generator (2-Level)1 : powerlib_meascontrol/Pulse & Signal Generators/PWM Generator (2-Level)  ModulatorType=Three-phase bridge (6 pulses)  ModulatorMode=Unsynchronized  Fc=fsw  Pc=0  nF=27  MinMax="[ -1  1 ]"  SamplingTechnique=Natural  ModulatingSignals=off  m=0.8  Freq=60  Phase=0  Ts=0  ShowCarrierOutport=off
  Vbus Control : Subsystem
  "abc - α/β  " : Subsystem
  "d/q  α/β " : Subsystem
  α/β - abc : Subsystem
  α/β - d/q : Subsystem
  PWM : Outport
  tag scope: P_SOC_ref=global, P_bat_ref=global, V_dc_bat_ref=global, f_ref=global, id_bat=global, id_bat_ref=global, iq_bat=global, iq_bat_ref=global
  wires:
  PWM Generator (2-Level)1/1 -> PWM/1
  PLL (3ph)/2 -> Manual Switch/2
  α/β - d/q/1(i d/q_bat) -> Demux/1
  Manual Switch/1 -> "d/q  α/β "/2(theta_bat (θ_bat)), α/β - d/q/2(theta_bat (θ_bat))
  " Angle Rotor"/1(theta_bat (θ_bat)) -> Manual Switch/1
  "V_ac_bat "/1 -> PLL (3ph)/1, " Angle Rotor"/1(Vabc_bat)
  α/β - abc/1(Vabc_bat) -> 3er Harmonic Inyection/1(in)
  i_ac_bat/1 -> "abc - α/β  "/1(iabc_bat)
  "d/q  α/β "/1("Vα/β_bat ") -> α/β - abc/1(V α/β_bat)
  "abc - α/β  "/1(i α/β_bat) -> α/β - d/q/1(i α/β_bat)
  3er Harmonic Inyection/1(out) -> Normalization/1
  PI Id1/1(out) -> Cancelation of cc/1(Id)
  PI Iq/1("out ") -> Cancelation of cc/2(Iq)
  Demux/2 -> [iq_bat], PI Iq/2(iq_bat_means)
  Gain1/1 -> [iq_bat_ref], PI Iq/1(iq_bat_ref)  "iq_bat_ref"
  Cancelation of cc/1(" Vdq_bat") -> "d/q  α/β "/1(Vdq_bat)
  Normalization/1 -> PWM Generator (2-Level)1/1
  Frequency Control/1("ΔP_bat_ref ") -> [P_bat_ref], Display11/1, Dischraging Control/1("Pot_ref ")  "ΔP_bat_ref"
  V_dc_bat/1 -> Display6/1, Vbus Control/2("means Vbus ")
  f_ref/1 -> Frequency Control/1(f_ref), [f_ref], Display5/1
  Q/1 -> Gain1/1
  [P_bat] -> Display12/1, Dischraging Control/2("Pot_means ")
  [Freq_mean] -> Display1/1, Frequency Control/2(f_means)
  Demux/1 -> PI Id1/2(idg_means), Display8/1, [id_bat_ref], [id_bat]
  [Freq_mean] -> Active Power Command/2(f), Display18/1
  [SOC] -> Active Power Command/1(SOC), Display17/1
  V_dc_bat_ref/1 -> [V_dc_bat_ref], Display7/1, Vbus Control/1("ref Vbus ")
  Active Power Command/1(Id*) -> Display2/1, PI Id1/1(idg_ref)
  Dischraging Control/1(Id*_P) -> Display10/1, Active Power Command/4(Id*_P)  "Id*_P"
  Charging Control/1(Id*_P) -> Display9/1, Active Power Command/3(Id*_SOC)
  Vbus Control/1(P_SOC_ref) -> [P_SOC_ref], Display4/1, Charging Control/1("Pot_ref ")  "P_SOC_ref"
  [P_bat] -> Charging Control/2("Pot_means "), Display3/1

== system Dfig2014a/BESS/Measurement of Power - Frequency ==
  PLL (3ph)1 : powerlib_meascontrol/PLL/PLL (3ph)  Fmin=45  Par_Init=[0, f]  ParK=[180, 3200, 1]  TcD=1e-4  MaxRateChangeFreq=12  FilterCutOffFreq=25  Ts=0  AGC=on
  "Power (3ph, Instantaneous)1" : powerlib_meascontrol/Measurements/Power (3ph, Instantaneous)
  F (Hz) : Outport
  P (W) : Outport  Port=2
  Q (VAR) : Outport  Port=3
  tag scope: Freq_mean=global, P_bat=global, Q_bat=global
  wires:
  [V_ac_bat] -> "Power (3ph, Instantaneous)1"/1, PLL (3ph)1/1
  "Power (3ph, Instantaneous)1"/1 -> P (W)/1, [P_bat]  "Pot"
  PLL (3ph)1/1 -> F (Hz)/1, [Freq_mean]
  [I_ac_bat] -> "Power (3ph, Instantaneous)1"/2
  "Power (3ph, Instantaneous)1"/2 -> Q (VAR)/1, [Q_bat]

== system Dfig2014a/BESS/Subsystem1 ==
  In1 : Inport
  Bus Selector : BusSelector  OutputSignals=SOC (%),Current (A),Voltage (V)
  tag scope: I_dc_bat=global, SOC=global, V_dc_bat=global
  wires:
  Bus Selector/3 -> [V_dc_bat]  "<Voltage (V)>"
  Bus Selector/1 -> [SOC]  "<SOC (%)>"
  In1/1 -> Bus Selector/1
  Bus Selector/2 -> [I_dc_bat]  "<Current (A)>"

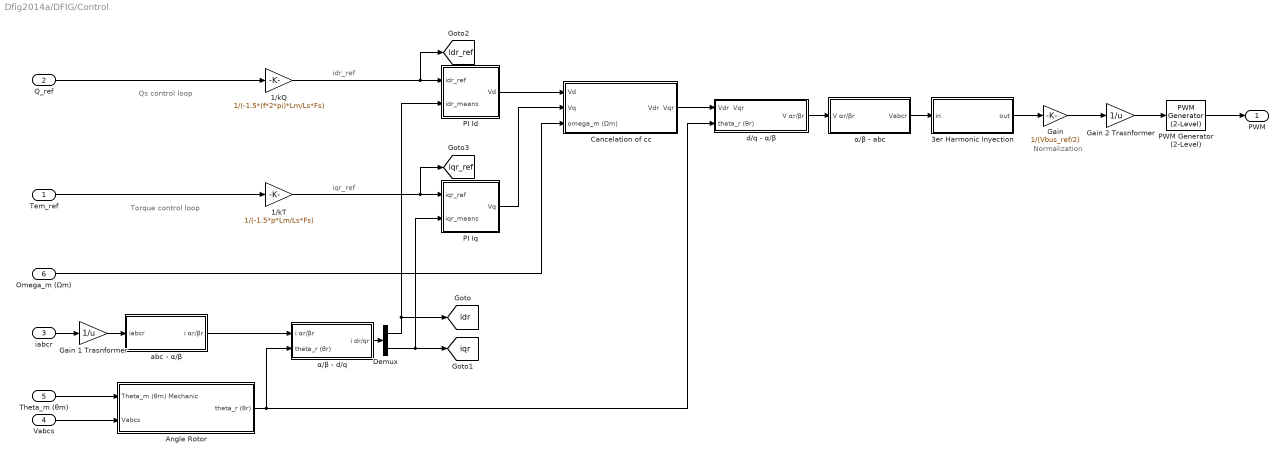
== system Dfig2014a/DFIG/Control ==
  note: Normalization
  note: Torque control loop
  note: iqr_ref
  note: idr_ref
  note: Qs control loop
  Tem_ref : Inport
  Q_ref : Inport  Port=2
  iabcr : Inport  Port=3
  Vabcs : Inport  Port=4
  Theta_m (θm) : Inport  Port=5
  "Omega_m (Ωm) " : Inport  Port=6
  " Angle Rotor" : Subsystem
  1/kQ : Gain  Gain=1/(-1.5*(f*2*pi)*Lm/Ls*Fs)
  1/kT : Gain  Gain=1/(-1.5*p*Lm/Ls*Fs)
  3er Harmonic Inyection : Subsystem
  Cancelation of cc : Subsystem
  Demux : Demux  Outputs=2
  Gain : Gain  Gain=1/(Vbus_ref/2)
  Gain 1 Trasnformer : Gain  Gain=1/u
  Gain 2 Trasnformer : Gain  Gain=1/u
  PI Id : Subsystem
  PI Iq : Subsystem
  PWM Generator (2-Level) : powerlib_meascontrol/Pulse & Signal Generators/PWM Generator (2-Level)  ModulatorType=Three-phase bridge (6 pulses)  ModulatorMode=Unsynchronized  Fc=fsw  Pc=0  nF=27  MinMax="[ -1  1 ]"  SamplingTechnique=Natural  ModulatingSignals=off  m=0.8  Freq=60  Phase=0  Ts=0  ShowCarrierOutport=off
  "abc - α/β " : Subsystem
  d/q - α/β : Subsystem
  α/β - abc : Subsystem
  α/β - d/q : Subsystem
  PWM : Outport
  tag scope: idr=global, idr_ref=global, iqr=global, iqr_ref=global
  wires:
  α/β - abc/1(Vabcr) -> 3er Harmonic Inyection/1(in)
  d/q - α/β/1(V αr/βr) -> α/β - abc/1(V αr/βr)
  iabcr/1 -> Gain 1 Trasnformer/1
  "abc - α/β "/1(i αr/βr) -> α/β - d/q/1(i αr/βr)
  3er Harmonic Inyection/1(out) -> Gain/1
  Theta_m (θm)/1 -> " Angle Rotor"/1(Theta_m (θm) Mechanic)
  Vabcs/1 -> " Angle Rotor"/2(Vabcs)
  " Angle Rotor"/1(theta_r (θr)) -> d/q - α/β/2(theta_r (θr)), α/β - d/q/2(theta_r (θr))
  PI Id/1(Vd) -> Cancelation of cc/1(Vd)
  PI Iq/1(Vq) -> Cancelation of cc/2(Vq)
  α/β - d/q/1(i dr/qr) -> Demux/1
  Demux/2 -> PI Iq/2(iqr_means), [iqr]
  Demux/1 -> PI Id/2(idr_means), [idr]
  1/kT/1 -> [iqr_ref], PI Iq/1(iqr_ref)
  Q_ref/1 -> 1/kQ/1
  Cancelation of cc/1(Vdr  Vqr) -> d/q - α/β/1(Vdr  Vqr)
  Gain/1 -> Gain 2 Trasnformer/1
  Gain 1 Trasnformer/1 -> "abc - α/β "/1(iabcr)
  Gain 2 Trasnformer/1 -> PWM Generator (2-Level)/1
  PWM Generator (2-Level)/1 -> PWM/1
  Tem_ref/1 -> 1/kT/1
  "Omega_m (Ωm) "/1 -> Cancelation of cc/3(omega_m (Ωm))
  1/kQ/1 -> [idr_ref], PI Id/1(idr_ref)

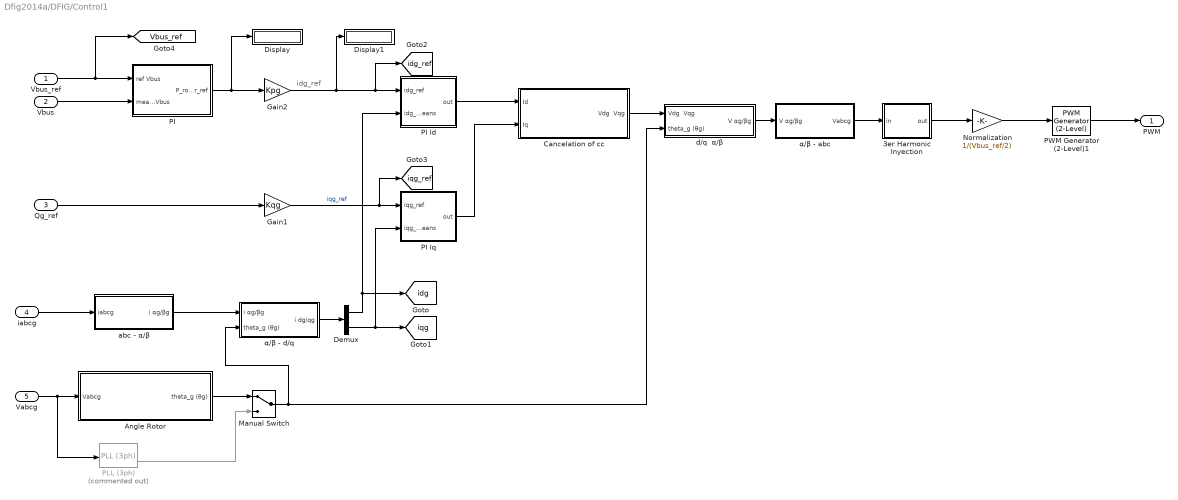
== system Dfig2014a/DFIG/Control1 ==
  note: idg_ref
  Vbus_ref : Inport
  Vbus : Inport  Port=2
  Qg_ref : Inport  Port=3
  iabcg : Inport  Port=4
  "Vabcg " : Inport  Port=5
  " Angle Rotor" : Subsystem
  3er Harmonic Inyection : Subsystem
  Cancelation of cc : Subsystem
  Demux : Demux  Outputs=2
  Display : Display
  Display1 : Display
  Gain1 : Gain  Gain=Kqg
  Gain2 : Gain  Gain=Kpg
  Manual Switch : ManualSwitch
  Normalization : Gain  Gain=1/(Vbus_ref/2)
  PI : Subsystem
  PI Id : Subsystem
  PI Iq : Subsystem
  PLL (3ph) : powerlib_meascontrol/PLL/PLL (3ph)  Commented=on  Fmin=45  Par_Init=[0, 60]  ParK=[180, 3200, 1]  TcD=1e-4  MaxRateChangeFreq=12  FilterCutOffFreq=25  Ts=0  AGC=on
      link override Model/abc to dq0: Alignment=Aligned with phase A axis
  PWM Generator (2-Level)1 : powerlib_meascontrol/Pulse & Signal Generators/PWM Generator (2-Level)  ModulatorType=Three-phase bridge (6 pulses)  ModulatorMode=Unsynchronized  Fc=fsw  Pc=0  nF=27  MinMax="[ -1  1 ]"  SamplingTechnique=Natural  ModulatingSignals=off  m=0.8  Freq=60  Phase=0  Ts=0  ShowCarrierOutport=off
  "abc - α/β  " : Subsystem
  "d/q  α/β " : Subsystem
  α/β - abc : Subsystem
  α/β - d/q : Subsystem
  PWM : Outport
  tag scope: Vbus_ref=global, idg=global, idg_ref=global, iqg=global, iqg_ref=global
  wires:
  Normalization/1 -> PWM Generator (2-Level)1/1
  Cancelation of cc/1(Vdg  Vqg) -> "d/q  α/β "/1(Vdg  Vqg)
  Gain1/1 -> PI Iq/1(iqg_ref), [iqg_ref]  "iqg_ref"
  Demux/1 -> PI Id/2(idg_means), [idg]
  Demux/2 -> PI Iq/2(iqg_means), [iqg]
  PI Iq/1(out) -> Cancelation of cc/2(Iq)
  PI Id/1(out) -> Cancelation of cc/1(Id)
  3er Harmonic Inyection/1(out) -> Normalization/1
  "abc - α/β  "/1(i αg/βg) -> α/β - d/q/1(i αg/βg)
  "d/q  α/β "/1(V αg/βg) -> α/β - abc/1(V αg/βg)
  iabcg/1 -> "abc - α/β  "/1(iabcg)
  Vbus_ref/1 -> [Vbus_ref], PI/1("ref Vbus ")
  Gain2/1 -> Display1/1, [idg_ref], PI Id/1(idg_ref)
  Vbus/1 -> PI/2("means Vbus ")
  Qg_ref/1 -> Gain1/1
  α/β - abc/1(Vabcg) -> 3er Harmonic Inyection/1(in)
  "Vabcg "/1 -> " Angle Rotor"/1("Vabcg "), PLL (3ph)/1
  PI/1(P_rotor_ref) -> Display/1, Gain2/1
  " Angle Rotor"/1(theta_g (θg)) -> Manual Switch/1
  Manual Switch/1 -> "d/q  α/β "/2(theta_g (θg)), α/β - d/q/2(theta_g (θg))
  α/β - d/q/1(i dg/qg) -> Demux/1
  PLL (3ph)/2 -> Manual Switch/2
  PWM Generator (2-Level)1/1 -> PWM/1

== system Dfig2014a/DFIG/MPPT ==
  note: Zone 2: MPPT with Vw 5 - 11
  Omega_m : Inport
  Display1 : Display
  Gearbox Ratio Generator Torque (-)1 : Gain  Gain=-1/N
  Gearbox Ratio1 : Gain  Gain=1/N
  Kopt : Gain  Gain=0.5*ro*pi*(Radio)^5/(lambda_opt)^3*cp_opt_abs
  Product2 : Product  Inputs=**  SaturateOnIntegerOverflow=on  InputSameDT=on  OutDataTypeStr=Inherit: Same as first input
  omega^2 : Fcn  Expr=(u[1])^2
  Tem_ref : Outport
  "Pot_ref " : Outport  Port=2
  wires:
  Gearbox Ratio1/1 -> Product2/2, omega^2/1
  omega^2/1 -> Kopt/1
  Kopt/1 -> Product2/1, Gearbox Ratio Generator Torque (-)1/1
  Product2/1 -> "Pot_ref "/1, Display1/1  "Pt"
  Gearbox Ratio Generator Torque (-)1/1 -> Tem_ref/1
  Omega_m/1 -> Gearbox Ratio1/1

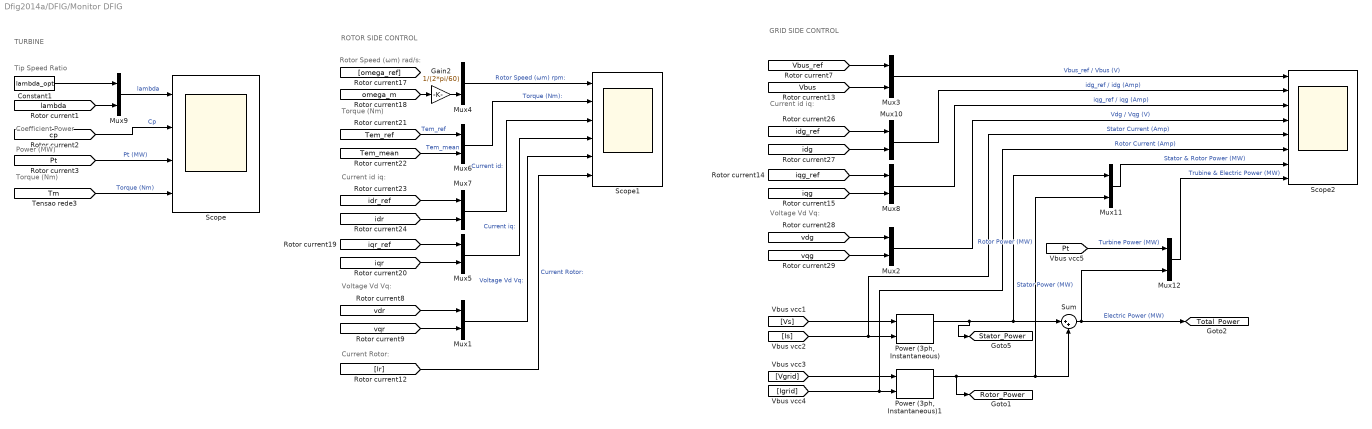
== system Dfig2014a/DFIG/Monitor DFIG ==
  note: ROTOR SIDE CONTROL
  note: Torque (Nm)
  note: Current id iq:
  note: Rotor Speed (ωm) rad/s:
  note: Voltage Vd Vq:
  note: TURBINE
  note: Torque (Nm)
  note: Power (MW)
  note: Coefficient Power
  note: Tip Speed Ratio
  note: GRID SIDE CONTROL
  note: Current id iq:
  note: Voltage Vd Vq:
  note: Current Rotor:
  Constant1 : Constant  Value=lambda_opt
  Gain2 : Gain  Gain=1/(2*pi/60)
  Mux{1..12} (12 alike) : Mux  Inputs=2
  "Power (3ph, Instantaneous)" : powerlib_meascontrol/Measurements/Power (3ph, Instantaneous)
  "Power (3ph, Instantaneous)1" : powerlib_meascontrol/Measurements/Power (3ph, Instantaneous)
  Scope : Scope  NumInputPorts=4
  Scope1 : Scope  NumInputPorts=6
  Scope2 : Scope  NumInputPorts=8
  Sum : Sum  Inputs=|++
  tag scope: Rotor_Power=global, Stator_Power=global, Total_Power=global
  wires:
  [iqr_ref] -> Mux5/1
  [iqr] -> Mux5/2
  [idr] -> Mux7/2
  [idr_ref] -> Mux7/1
  [vdr] -> Mux1/1
  [vqr] -> Mux1/2
  [vqg] -> Mux2/2
  [vdg] -> Mux2/1
  [idg_ref] -> Mux10/1
  [idg] -> Mux10/2
  [iqg] -> Mux8/2
  [iqg_ref] -> Mux8/1
  [Tem_ref] -> Mux6/1  "Tem_ref"
  [Vbus] -> Mux3/2
  [Vbus_ref] -> Mux3/1
  [cp] -> Scope/2  "Cp"
  [Pt] -> Scope/3  "Pt (MW)"
  [Tm] -> Scope/4  "Torque (Nm)"
  Mux4/1 -> Scope1/1  "Rotor Speed (ωm) rpm:"
  Mux6/1 -> Scope1/2  "Torque (Nm):"
  Mux7/1 -> Scope1/3  "Current id:"
  Mux5/1 -> Scope1/4  "Current iq:"
  Mux1/1 -> Scope1/5  "Voltage Vd Vq:"
  [Ir] -> Scope1/6  "Current Rotor:"
  [omega_m] -> Gain2/1
  Gain2/1 -> Mux4/2
  Mux3/1 -> Scope2/1  "Vbus_ref / Vbus (V)"
  Mux10/1 -> Scope2/2  "idg_ref / idg (Amp)"
  Mux8/1 -> Scope2/3  "iqg_ref / iqg (Amp)"
  Mux2/1 -> Scope2/4  "Vdg / Vqg (V)"
  [lambda] -> Mux9/2
  Constant1/1 -> Mux9/1
  Mux9/1 -> Scope/1  "lambda"
  [Tem_mean] -> Mux6/2  "Tem_mean"
  [Vs] -> "Power (3ph, Instantaneous)"/1
  [Vgrid] -> "Power (3ph, Instantaneous)1"/1
  [Igrid] -> "Power (3ph, Instantaneous)1"/2, Scope2/6  "Rotor Current (Amp)"
  [Is] -> "Power (3ph, Instantaneous)"/2, Scope2/5  "Stator Current (Amp)"
  "Power (3ph, Instantaneous)"/1 -> [Stator_Power], Mux11/1, Sum/1  "Stator Power (MW)"
  "Power (3ph, Instantaneous)1"/1 -> [Rotor_Power], Sum/2, Mux11/2  "Rotor Power (MW)"
  Sum/1 -> [Total_Power], Mux12/2  "Electric Power (MW)"
  Mux11/1 -> Scope2/7  "Stator & Rotor Power (MW)"
  [Pt] -> Mux12/1  "Turbine Power (MW)"
  Mux12/1 -> Scope2/8  "Trubine & Electric Power (MW)"

== system Dfig2014a/DFIG/Subsystem ==
  In1 : Inport
  Bus Selector : BusSelector  OutputSignals=Mechanical.Rotor angle thetam (rad),Mechanical.Rotor speed (wm),Mechanical.Electromagnetic torque Te (N*m)
  tag scope: Tem_mean=global, omega_m=global, tita_m=global
  wires:
  Bus Selector/2 -> [omega_m]  "<Rotor speed (wm)>"
  In1/1 -> Bus Selector/1
  Bus Selector/1 -> [tita_m]  "<Rotor angle thetam (rad)>"
  Bus Selector/3 -> [Tem_mean]  "<Electromagnetic torque Te (N*m)>"

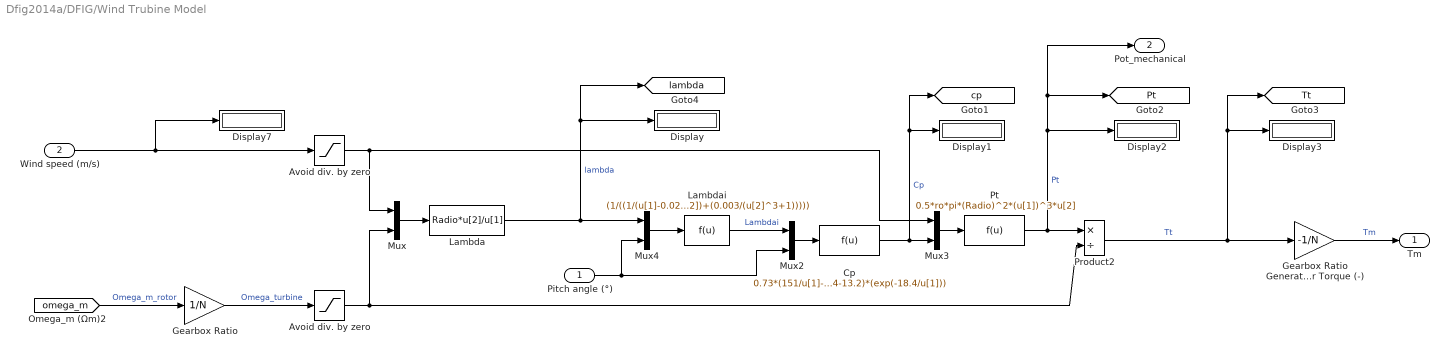
== system Dfig2014a/DFIG/Wind Trubine Model ==
  Pitch angle (°) : Inport
  Wind speed (m/s) : Inport  Port=2
  Avoid div. by zero : Saturate  UpperLimit=inf  LowerLimit=eps
  "Avoid div. by zero " : Saturate  UpperLimit=inf  LowerLimit=eps
  Cp : Fcn  Expr=0.73*(151/u[1]-0.58*u[2]-0.002*u[2]^2.14-13.2)*(exp(-18.4/u[1]))
  Display{,1..3,7} (5 alike) : Display
  Gearbox Ratio : Gain  Gain=1/N
  Gearbox Ratio Generator Torque (-) : Gain  Gain=-1/N
  Lambda : Fcn  Expr=Radio*u[2]/u[1]
  Lambdai : Fcn  Expr=(1/((1/(u[1]-0.02*u[2])+(0.003/(u[2]^3+1)))))
  Mux{,2..4} (4 alike) : Mux  Inputs=2
  Product2 : Product  Inputs=*/  SaturateOnIntegerOverflow=on  InputSameDT=on  OutDataTypeStr=Inherit: Same as first input
  Pt : Fcn  Expr=0.5*ro*pi*(Radio)^2*(u[1])^3*u[2]
  Tm : Outport
  Pot_mechanical : Outport  Port=2
  tag scope: Pt=global, Tt=global, cp=global, lambda=global
  wires:
  "Avoid div. by zero "/1 -> Product2/2, Mux/2
  Avoid div. by zero/1 -> Mux/1, Mux3/1
  [omega_m] -> Gearbox Ratio/1  "Omega_m_rotor"
  Mux3/1 -> Pt/1
  Cp/1 -> Display1/1, [cp], Mux3/2  "Cp"
  Mux/1 -> Lambda/1
  Mux2/1 -> Cp/1
  Product2/1 -> Display3/1, [Tt], Gearbox Ratio Generator Torque (-)/1  "Tt"
  Pt/1 -> Display2/1, Pot_mechanical/1, [Pt], Product2/1  "Pt"
  Gearbox Ratio/1 -> "Avoid div. by zero "/1  "Omega_turbine"
  Wind speed (m/s)/1 -> Display7/1, Avoid div. by zero/1
  Lambdai/1 -> Mux2/1  "Lambdai"
  Mux4/1 -> Lambdai/1
  Gearbox Ratio Generator Torque (-)/1 -> Tm/1  "Tm"
  Pitch angle (°)/1 -> Mux2/2, Mux4/2
  Lambda/1 -> Display/1, [lambda], Mux4/1  "lambda"

== system Dfig2014a/BESS/Control System/ Angle Rotor ==
  note: V α/β_bat
  Vabc_bat : Inport
  " abc - αβ " : Subsystem
  Demux : Demux  Outputs=2
  θv=tan^(-1) (Vβ/Vα) : Trigonometry  Operator=atan2
  theta_bat (θ_bat) : Outport
  wires:
  θv=tan^(-1) (Vβ/Vα)/1 -> theta_bat (θ_bat)/1
  Vabc_bat/1 -> " abc - αβ "/1(Vabc_bat)
  Demux/2 -> θv=tan^(-1) (Vβ/Vα)/1
  Demux/1 -> θv=tan^(-1) (Vβ/Vα)/2
  " abc - αβ "/1("V α/β_bat ") -> Demux/1

== system Dfig2014a/BESS/Control System/3er Harmonic Inyection ==
  in : Inport
  Gain : Gain  Gain=-0.5
  MinMax : MinMax
  MinMax1 : MinMax  Function=max
  Scope : Scope
  Sum : Sum  Inputs=|++
  Sum1 : Sum  Inputs=|++
  out : Outport
  wires:
  in/1 -> Sum1/1, MinMax1/1, MinMax/1
  MinMax/1 -> Sum/1
  MinMax1/1 -> Sum/2
  Sum1/1 -> out/1
  Sum/1 -> Gain/1
  Gain/1 -> Scope/1, Sum1/2
